simulink model "polyphase_filter"  (R2019b)
settings: Solver=FixedStepDiscrete  StartTime=0.0  StopTime=1  FixedStep=5 ns  RelTol=1e-3
undefined symbols (not defined in the file or in its folder): designMultirateFIR
libraries: dspsrcs4 x3, dspmlti4 x1, commfilt2 x1
settings Model: Creator=thomas  LastModifiedBy=thomas

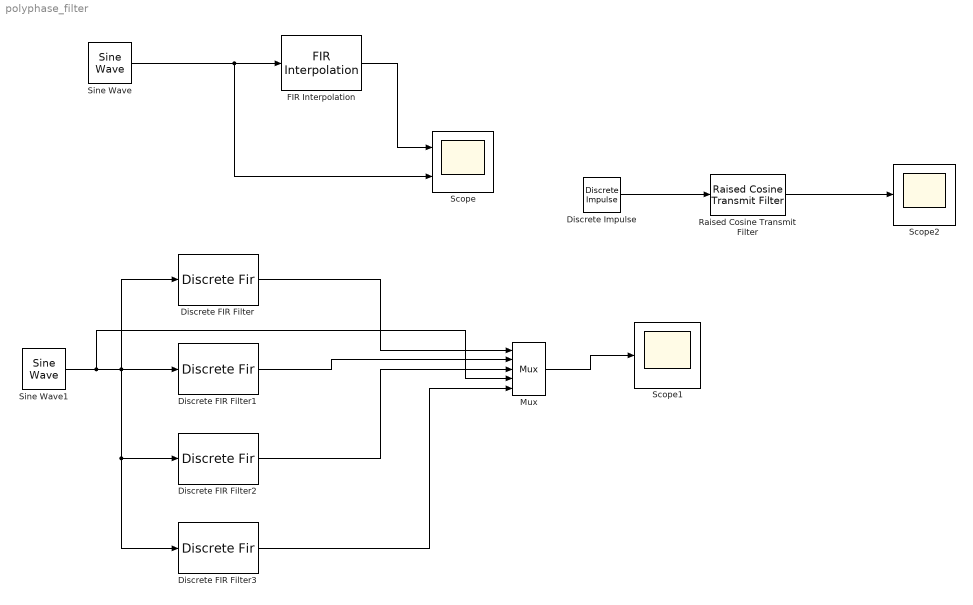
== system polyphase_filter ==
  Discrete Impulse : dspsrcs4/Discrete  Impulse  Delay=0  SampleTime=1  FrameSample=1  OutputFrames=off  dataType=double  isSigned=on  wordLen=16  udDataType=sfix(16)  fracBitsMode=Best precision  numFracBits=15  OutDataTypeStr=double  LastOutDataTypeStr=double
  Discrete FIR Filter : DiscreteFir  Coefficients="[0\t0\t0\t0\t0\t0\t0\t0\t0\t0\t0\t0\t0\t0\t0\t0\t0\t0\t0\t0\t0\t0\t0\t0\t0\t1\t0\t0\t0\t0\t0\t0\t0\t0\t0\t0\t0\t0\t0\t0\t0\t0\t0\t0\t0\t0\t0\t0\t0\t0\t0]"  InputProcessing=Columns as channels (frame based)
  Discrete FIR Filter1 : DiscreteFir  Coefficients="[-0.000713121834579885\t0.000776195528888330\t-0.000914370407591774\t0.00113604559592819\t-0.00145002750358115\t0.00186567973686579\t-0.00239313935165103\t0.00304362370295496\t-0.00382986307092910\t0.00476671124333886\t-0.00587201330167646\t0.00716785406117838\t-0.00868238489203801\t0.0104525555545236\t-0.0125283097769446\t0.0149792392694490\t-0.0179055510981797\t0.0214570021077444\t-0.0258674859011711\t0.0315227956549018\t-0.0391057887030259\t0.0499464284497222\t-0.0670179664163128\t0.0985894637270710\t-0.179410131029501\t0.900316316157106\t0.299016885049169\t-0.126757881934806\t0.0792030512192788\t-0.0566059522430185\t0.0432221875138708\t-0.0342639083205455\t0.0277835959679246\t-0.0228413248243732\t0.0189287254466471\t-0.0157474053858311\t0.0131110218595932\t-0.0108973451525885\t0.00902287057407875\t-0.00742850329976671\t0.00607106460003839\t-0.00491803540979408\t0.00394418734170312\t-0.00312935958191145\t0.00245695640102840\t-0.00191291213526746\t0.00148496792535419\t-0.00116216158663919\t0.000934466460505891\t-0.000792536487391247\t0.000727528336288568]"  InputProcessing=Columns as channels (frame based)
  Discrete FIR Filter2 : DiscreteFir  Coefficients="[-0.000998619250772677\t0.00108650515988472\t-0.00127935848856116\t0.00158875985491102\t-0.00202680381066476\t0.00260629312854320\t-0.00334102025432091\t0.00424616724489159\t-0.00533886937841210\t0.00663900908690910\t-0.00817034083596178\t0.00996210269493941\t-0.0120513622742104\t0.0144865029101323\t-0.0173325380871194\t0.0206794661067701\t-0.0246558975941573\t0.0294522897595626\t-0.0353627444064000\t0.0428653510952671\t-0.0527901214442470\t0.0667107544776003\t-0.0880078800979988\t0.125483901038923\t-0.211436867107546\t0.636619772367581\t0.634310601322637\t-0.209139835064871\t0.123211032137198\t-0.0857709700426290\t0.0645212595429685\t-0.0506590512944066\t0.0408031666227692\t-0.0333792617275043\t0.0275565914287640\t-0.0228562520127459\t0.0189832560001783\t-0.0157461988153612\t0.0130154712561472\t-0.0107000362278979\t0.00873381261775224\t-0.00706733225380646\t0.00566243721952798\t-0.00448880537317110\t0.00352161594374366\t-0.00273994918641721\t0.00212567228923378\t-0.00166265566211619\t0.00133621886583054\t-0.00113273942200747\t0.00103937922019197]"  InputProcessing=Columns as channels (frame based)
  Discrete FIR Filter3 : DiscreteFir  Coefficients="[-0.000699274808665719\t0.000760514811133012\t-0.000895120504274061\t0.00111107756085285\t-0.00141669353798160\t0.00182072359862806\t-0.00233255354528012\t0.00296246040420952\t-0.00372197960414237\t0.00462442135547803\t-0.00568560018098832\t0.00692487595740967\t-0.00836666180505481\t0.0100426514151306\t-0.0119951902119682\t0.0142825304662189\t-0.0169873177085295\t0.0202308877015877\t-0.0241986158430311\t0.0291877737545388\t-0.0357052853375455\t0.0446889096655409\t-0.0580822375608045\t0.0806641066857855\t-0.128150093592501\t0.300105438719035\t0.897050655147506\t-0.177461034708728\t0.0968037292680073\t-0.0653145602804059\t0.0483071507507968\t-0.0375271376844069\t0.0300062836453585\t-0.0244165886053644\t0.0200759209282620\t-0.0165986164877678\t0.0137505839015245\t-0.0113816716038146\t0.00939115100567374\t-0.00770882417900319\t0.00628408441056601\t-0.00507928247241027\t0.00406554695221703\t-0.00322006565674946\t0.00252427027502916\t-0.00196259816475493\t0.00152163380005429\t-0.00118950656514834\t0.000955465706809392\t-0.000809580282819008\t0.000742528920541939]"  InputProcessing=Columns as channels (frame based)
  FIR Interpolation : dspmlti4/FIR Interpolation  FilterSource=Auto  h=designMultirateFIR(3,1)  L=3  FilterObject=FINTERP  InputProcessing=Columns as channels (frame based)  framing=Enforce single-rate processing  outputBufInitCond=0  roundingMode=Floor  overflowMode=off  firstCoeffDataTypeStr=Inherit: Same word length as input  firstCoeffMin=[]  firstCoeffMax=[]  firstCoeffLastDataTypeStr=Inherit: Same word length as input  outputDataTypeStr=Inherit: Same as accumulator  outputMin=[]  outputMax=[]  outputLastDataTypeStr=Inherit: Same as accumulator
      settings: SourceProductName=DSP System Toolbox
  Mux : Mux  Inputs=5
  Raised Cosine Transmit Filter : commfilt2/Raised Cosine Transmit Filter  filtType=Square root  R=0.2  filtSpan=100  N=8  filterGain=1  RateOptions=Allow multirate processing  framing=Mute  checkCoeff=on  variableName=rcTxFilt  checkGain=Normalized  sampMode=Mute  saveAsFlag=0  currentFiltSpan=100  D=(100)/2  launchFVT=on  roundingMode=Floor  overflowMode=off  coeffMode=Binary point scaling  coeffWordLength=32  coeffFracLength=0  coeffDataTypeStr=fixdt(1,32,0)  coeffMin=[]  coeffMax=[]  coeffLastDataTypeStr=fixdt(1,32,0)  prodOutputMode=Binary point scaling  prodOutputWordLength=32  prodOutputFracLength=5  prodOutputDataTypeStr=fixdt(1,32,5)  prodOutputLastDataTypeStr=fixdt(1,32,5)  accumMode=Binary point scaling  accumWordLength=64  accumFracLength=0  accumDataTypeStr=fixdt(1,64,0)  accumLastDataTypeStr=fixdt(1,64,0)  outputMode=Binary point scaling  outputWordLength=64  outputFracLength=0  outputDataTypeStr=fixdt(1,64,0)  outputMin=[]  outputMax=[]  outputLastDataTypeStr=fixdt(1,64,0)
      settings: SourceProductName=Communications Toolbox
  Scope : Scope  NumInputPorts=2
  Scope1 : Scope
  Scope2 : Scope
  Sine Wave : dspsrcs4/Sine Wave  Amplitude=1  Frequency=100  Phase=0  SampleMode=Discrete  OutComplex=Real  CompMethod=Trigonometric fcn  TableSize=Speed  SampleTime=1/10000  SamplesPerFrame=1  ResetState=Restart at time zero  OutputFrames=off  dataType=double  wordLen=16  udDataType=sfix(16)  fracBitsMode=Best precision  numFracBits=15  OutDataTypeStr=double  LastOutDataTypeStr=double
  Sine Wave1 : dspsrcs4/Sine Wave  Amplitude=10  Frequency=10  Phase=0  SampleMode=Discrete  OutComplex=Real  CompMethod=Trigonometric fcn  TableSize=Speed  SampleTime=1/10000  SamplesPerFrame=1  ResetState=Restart at time zero  OutputFrames=off  dataType=double  wordLen=16  udDataType=sfix(16)  fracBitsMode=Best precision  numFracBits=15  OutDataTypeStr=double  LastOutDataTypeStr=double
  wires:
  Sine Wave/1 -> Scope/2, FIR Interpolation/1
  FIR Interpolation/1 -> Scope/1
  Sine Wave1/1 -> Mux/4, Discrete FIR Filter/1, Discrete FIR Filter1/1, Discrete FIR Filter3/1, Discrete FIR Filter2/1
  Discrete FIR Filter2/1 -> Mux/3
  Mux/1 -> Scope1/1
  Discrete FIR Filter1/1 -> Mux/2
  Discrete FIR Filter/1 -> Mux/1
  Discrete FIR Filter3/1 -> Mux/5
  Raised Cosine Transmit Filter/1 -> Scope2/1
  Discrete Impulse/1 -> Raised Cosine Transmit Filter/1
